simulink model "neuronchainv6"  (Simulink 7.6)
settings: Solver=ode45  StartTime=0.0  StopTime=300  RelTol=1e-3
values from neighbouring files (symbols this model uses):
  alpha = 0.8    [excneuroninit.m]
  beta = 0.05    [excneuroninit.m]
  inittime = 0.1    [excneuroninit.m]
  sensoryamp = 0.5    [excneuroninit.m]
  sigslopef = 1    [excneuroninit.m]
  sigslopei = 3    [excneuroninit.m]
  tau_s = 5    [excneuroninit.m]
libraries: simulink x500, neuronpoolibv3 x3
(part 18 of 18)

== system neuronchainv6/Hebbconp51to2/5/f(uj) ==
  x : Inport
  Constant : Constant  Value=offset
  Constant1 : Constant  Value=slope
  Constant2 : Constant
  Gain : Gain  Gain=-1  SaturateOnIntegerOverflow=on  OutDataTypeStr=Inherit: Same as input  ParamDataTypeStr=Inherit: Same as input
  Math Function : Math  SaturateOnIntegerOverflow=on
  Math Function1 : Math  Operator=reciprocal  SaturateOnIntegerOverflow=on
  Model Info : simulink/Model-Wide Utilities/Model Info  SystemSampleTime=-1  InitialBlockCM=None  BlockCM=None  Frame=on  DisplayStringWithTags=|  HorizontalTextAlignment=Center  LeftAlignmentValue=0.5  SourceBlockDiagram=neuronchainv6  TagMaxNumber=20
      | Model Info
      | %<Creator> Han, Cheol
  Product : Product  SaturateOnIntegerOverflow=on  OutDataTypeStr=Inherit: Same as first input
  Sum : Sum  Inputs=+-  SaturateOnIntegerOverflow=on
  Sum1 : Sum  SaturateOnIntegerOverflow=on
  y : Outport  InitialOutput=0
  wires:
  x/1 -> Sum/1
  Constant/1 -> Sum/2
  Sum/1 -> Product/1
  Constant1/1 -> Product/2
  Product/1 -> Gain/1
  Gain/1 -> Math Function/1
  Math Function/1 -> Sum1/1
  Constant2/1 -> Sum1/2
  Sum1/1 -> Math Function1/1
  Math Function1/1 -> y/1

== system neuronchainv6/Hebbconp51to2/5/h(ui) ==
  x : Inport
  Constant : Constant  Value=offset
  Constant1 : Constant  Value=slope
  Constant2 : Constant
  Gain : Gain  Gain=-1  SaturateOnIntegerOverflow=on  OutDataTypeStr=Inherit: Same as input  ParamDataTypeStr=Inherit: Same as input
  Math Function : Math  SaturateOnIntegerOverflow=on
  Math Function1 : Math  Operator=reciprocal  SaturateOnIntegerOverflow=on
  Model Info : simulink/Model-Wide Utilities/Model Info  SystemSampleTime=-1  InitialBlockCM=None  BlockCM=None  Frame=on  DisplayStringWithTags=|  HorizontalTextAlignment=Center  LeftAlignmentValue=0.5  SourceBlockDiagram=neuronchainv6  TagMaxNumber=20
      | Model Info
      | %<Creator> Han, Cheol
  Product : Product  SaturateOnIntegerOverflow=on  OutDataTypeStr=Inherit: Same as first input
  Sum : Sum  Inputs=+-  SaturateOnIntegerOverflow=on
  Sum1 : Sum  SaturateOnIntegerOverflow=on
  y : Outport  InitialOutput=0
  wires:
  x/1 -> Sum/1
  Constant/1 -> Sum/2
  Sum/1 -> Product/1
  Constant1/1 -> Product/2
  Product/1 -> Gain/1
  Gain/1 -> Math Function/1
  Math Function/1 -> Sum1/1
  Constant2/1 -> Sum1/2
  Sum1/1 -> Math Function1/1
  Math Function1/1 -> y/1

== system neuronchainv6/Subsystem/motoract vis inputs/Subsystem ==
  Saturation : Saturate  UpperLimit=1  LowerLimit=0
  Signal Generator : SignalGenerator  WaveForm=square
  Signal Generator1 : SignalGenerator  WaveForm=square  Frequency=0.5
  Sum : Sum  Inputs=|+-
  Tapped Delay{,1..3} (4 alike) : simulink/Discrete/Tapped Delay  vinit=0.0  samptime=-1  NumDelays=1  DelayOrder=Oldest  includeCurrent=off
  Out1 : Outport
  Out2 : Outport  Port=2
  wires:
  Signal Generator/1 -> Sum/1
  Signal Generator1/1 -> Sum/2
  Sum/1 -> Saturation/1
  Saturation/1 -> Tapped Delay/1, Out1/1
  Tapped Delay1/1 -> Tapped Delay2/1
  Tapped Delay/1 -> Tapped Delay1/1
  Tapped Delay2/1 -> Tapped Delay3/1
  Tapped Delay3/1 -> Out2/1

== system neuronchainv6/Subsystem/motoract vis inputs/Subsystem1 ==
  Saturation1 : Saturate  UpperLimit=1  LowerLimit=0
  Signal Generator2 : SignalGenerator  WaveForm=square
  Signal Generator3 : SignalGenerator  WaveForm=square  Frequency=0.5
  Sum1 : Sum  Inputs=|+-
  Tapped Delay{3..6} (4 alike) : simulink/Discrete/Tapped Delay  vinit=0.0  samptime=-1  NumDelays=1  DelayOrder=Oldest  includeCurrent=off
  Out1 : Outport
  Out2 : Outport  Port=2
  wires:
  Signal Generator2/1 -> Sum1/1
  Signal Generator3/1 -> Sum1/2
  Sum1/1 -> Saturation1/1
  Saturation1/1 -> Tapped Delay3/1, Out1/1
  Tapped Delay4/1 -> Tapped Delay5/1
  Tapped Delay3/1 -> Tapped Delay4/1
  Tapped Delay5/1 -> Tapped Delay6/1
  Tapped Delay6/1 -> Out2/1

== system neuronchainv6/Subsystem/motoract vis inputs/Subsystem2 ==
  Saturation : Saturate  UpperLimit=1  LowerLimit=0
  Signal Generator : SignalGenerator  WaveForm=square
  Signal Generator1 : SignalGenerator  WaveForm=square  Frequency=0.5
  Sum : Sum  Inputs=|+-
  Tapped Delay{,1..3} (4 alike) : simulink/Discrete/Tapped Delay  vinit=0.0  samptime=-1  NumDelays=1  DelayOrder=Oldest  includeCurrent=off
  Out1 : Outport
  Out2 : Outport  Port=2
  wires:
  Signal Generator/1 -> Sum/1
  Signal Generator1/1 -> Sum/2
  Sum/1 -> Saturation/1
  Saturation/1 -> Tapped Delay/1, Out1/1
  Tapped Delay1/1 -> Tapped Delay2/1
  Tapped Delay/1 -> Tapped Delay1/1
  Tapped Delay2/1 -> Tapped Delay3/1
  Tapped Delay3/1 -> Out2/1

== system neuronchainv6/Subsystem/motoract vis inputs/Subsystem3 ==
  Saturation1 : Saturate  UpperLimit=1  LowerLimit=0
  Signal Generator2 : SignalGenerator  WaveForm=square
  Signal Generator3 : SignalGenerator  WaveForm=square  Frequency=0.5
  Sum1 : Sum  Inputs=|+-
  Tapped Delay{3..6} (4 alike) : simulink/Discrete/Tapped Delay  vinit=0.0  samptime=-1  NumDelays=1  DelayOrder=Oldest  includeCurrent=off
  Out1 : Outport
  Out2 : Outport  Port=2
  wires:
  Signal Generator2/1 -> Sum1/1
  Signal Generator3/1 -> Sum1/2
  Sum1/1 -> Saturation1/1
  Saturation1/1 -> Tapped Delay3/1, Out1/1
  Tapped Delay4/1 -> Tapped Delay5/1
  Tapped Delay3/1 -> Tapped Delay4/1
  Tapped Delay5/1 -> Tapped Delay6/1
  Tapped Delay6/1 -> Out2/1

== system neuronchainv6/Subsystem/motoract vis inputs/Subsystem4 ==
  Saturation1 : Saturate  UpperLimit=1  LowerLimit=0
  Signal Generator2 : SignalGenerator  WaveForm=square
  Signal Generator3 : SignalGenerator  WaveForm=square  Frequency=0.5
  Sum1 : Sum  Inputs=|+-
  Tapped Delay{3..6} (4 alike) : simulink/Discrete/Tapped Delay  vinit=0.0  samptime=-1  NumDelays=1  DelayOrder=Oldest  includeCurrent=off
  Out1 : Outport
  Out2 : Outport  Port=2
  wires:
  Signal Generator2/1 -> Sum1/1
  Signal Generator3/1 -> Sum1/2
  Sum1/1 -> Saturation1/1
  Saturation1/1 -> Tapped Delay3/1, Out1/1
  Tapped Delay4/1 -> Tapped Delay5/1
  Tapped Delay3/1 -> Tapped Delay4/1
  Tapped Delay5/1 -> Tapped Delay6/1
  Tapped Delay6/1 -> Out2/1
